simulink library "bh_4bar_SL_LIB"  (R2019a)
settings: Solver=VariableStepAuto  StartTime=0.0  StopTime=10.0  RelTol=1e-3
settings Model: Creator=bhorton  LastModifiedBy=bhorton

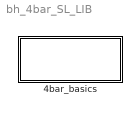
== system bh_4bar_SL_LIB ==
  4bar_basics : Subsystem

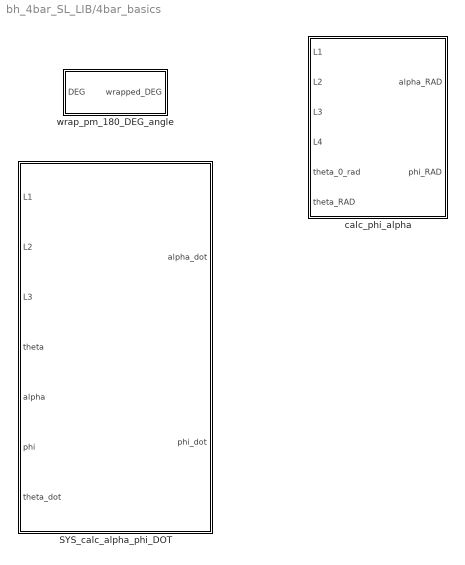
== system bh_4bar_SL_LIB/4bar_basics ==
  SYS_calc_alpha_phi_DOT : Subsystem
  calc_phi_alpha : Subsystem
  wrap_pm_180_DEG_angle : Subsystem

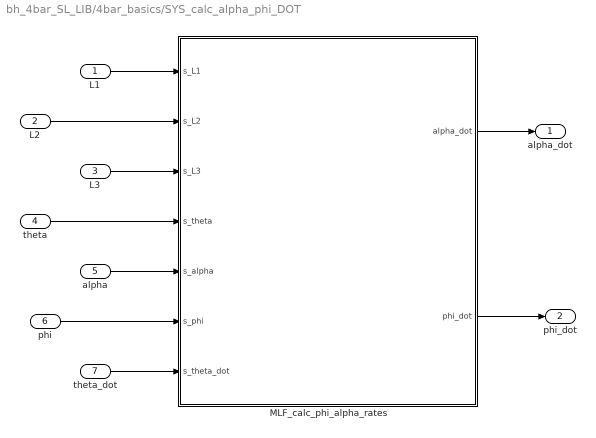
== system bh_4bar_SL_LIB/4bar_basics/SYS_calc_alpha_phi_DOT ==
  L1 : Inport
  L2 : Inport  Port=2
  L3 : Inport  Port=3
  theta : Inport  Port=4
  alpha : Inport  Port=5
  phi : Inport  Port=6
  theta_dot : Inport  Port=7
  MLF_calc_phi_alpha_rates : MATLAB Function  TreatAsAtomicUnit=on
  alpha_dot : Outport
  phi_dot : Outport  Port=2
  wires:
  theta_dot/1 -> MLF_calc_phi_alpha_rates/7(s_theta_dot)
  phi/1 -> MLF_calc_phi_alpha_rates/6(s_phi)
  alpha/1 -> MLF_calc_phi_alpha_rates/5(s_alpha)
  theta/1 -> MLF_calc_phi_alpha_rates/4(s_theta)
  L3/1 -> MLF_calc_phi_alpha_rates/3(s_L3)
  L2/1 -> MLF_calc_phi_alpha_rates/2(s_L2)
  L1/1 -> MLF_calc_phi_alpha_rates/1(s_L1)
  MLF_calc_phi_alpha_rates/2(phi_dot) -> phi_dot/1
  MLF_calc_phi_alpha_rates/1(alpha_dot) -> alpha_dot/1

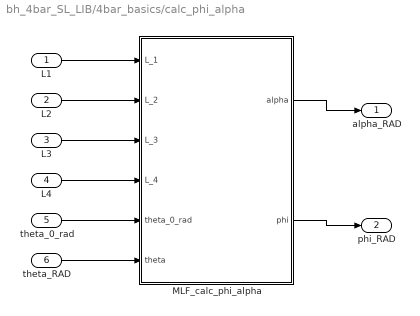
== system bh_4bar_SL_LIB/4bar_basics/calc_phi_alpha ==
  L1 : Inport
  L2 : Inport  Port=2
  L3 : Inport  Port=3
  L4 : Inport  Port=4
  theta_0_rad : Inport  Port=5
  theta_RAD : Inport  Port=6
  MLF_calc_phi_alpha : MATLAB Function  TreatAsAtomicUnit=on
  alpha_RAD : Outport
  phi_RAD : Outport  Port=2
  wires:
  theta_0_rad/1 -> MLF_calc_phi_alpha/5(theta_0_rad)
  MLF_calc_phi_alpha/2(phi) -> phi_RAD/1
  MLF_calc_phi_alpha/1(alpha) -> alpha_RAD/1
  L1/1 -> MLF_calc_phi_alpha/1(L_1)
  L2/1 -> MLF_calc_phi_alpha/2(L_2)
  L3/1 -> MLF_calc_phi_alpha/3(L_3)
  L4/1 -> MLF_calc_phi_alpha/4(L_4)
  theta_RAD/1 -> MLF_calc_phi_alpha/6(theta)

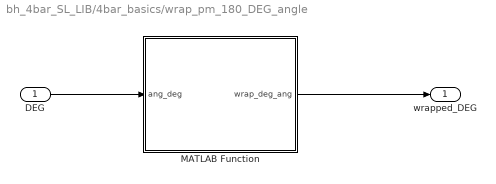
== system bh_4bar_SL_LIB/4bar_basics/wrap_pm_180_DEG_angle ==
  DEG : Inport
  MATLAB Function : MATLAB Function  TreatAsAtomicUnit=on
  wrapped_DEG : Outport
  wires:
  DEG/1 -> MATLAB Function/1(ang_deg)
  MATLAB Function/1(wrap_deg_ang) -> wrapped_DEG/1

== matlab function bh_4bar_SL_LIB/4bar_basics/calc_phi_alpha/MLF_calc_phi_alpha ==
  data: alpha output; L_1 input; phi output; L_2 input; L_3 input; L_4 input; theta_0_rad input; theta input
function [alpha, phi] = calc_phi_alpha(L_1, L_2, L_3, L_4, theta_0_rad, theta)

% Out of the 2 solution scenarios we'll choose the solution that covers the
% situation where phi is POSITIVE when theta==0

[phi_pair_rad, alpha_pair_rad] = bh_angle_calc_util(L_1, L_2, L_3, L_4, theta, "CALC_PHI_AND_ALPHA_VEC");          

[phi_pair_rad_ZERO, alpha_pair_rad_ZERO] = bh_angle_calc_util(L_1, L_2, L_3, L_4, theta_0_rad, "CALC_PHI_AND_ALPHA_VEC");          

if( phi_pair_rad_ZERO(1) >=0 )
  alpha = alpha_pair_rad(1);
  phi   =   phi_pair_rad(1);
else
  alpha = alpha_pair_rad(2);
  phi   =   phi_pair_rad(2);
end
    
% [phi, alpha] = bh_angle_calc_util(L_1, L_2, L_3, L_4, theta, ...
%                 "CALC_PHI_AND_ALPHA_VAL_AND_PHI_IS_POS");
            
end

== matlab function bh_4bar_SL_LIB/4bar_basics/wrap_pm_180_DEG_angle/MATLAB Function ==
  data: ang_deg input; wrap_deg_ang output
function wrap_deg_ang = wrap_to_pm_180(ang_deg)
%#codegen
   wrap_deg_ang = bh_wrap_DEG_angles(ang_deg, "-180_TO_180");
end

== matlab function bh_4bar_SL_LIB/4bar_basics/SYS_calc_alpha_phi_DOT/MLF_calc_phi_alpha_rates ==
  data: alpha_dot output; s_L1 input; phi_dot output; s_L2 input; s_L3 input; s_theta input; s_alpha input; s_phi input; s_theta_dot input
function [alpha_dot, phi_dot ] = ...
       calc_phi_alpha_rates(s_L1, s_L2, s_L3, s_theta, s_alpha, s_phi, s_theta_dot)

   k = 1/( s_L3*s_L2*(sin(s_phi)*cos(s_alpha)   -  cos(s_phi)*sin(s_alpha))  );
       
   tmp_A      =   [-s_L2*cos(s_alpha), -s_L2*sin(s_alpha);
                   -s_L3*cos(s_phi),   -s_L3*sin(s_phi);   ];
               
   tmp_B      =   [ -s_L1*sin(s_theta);
                     s_L1*cos(s_theta); ];
   
   the_jacobs    = k * tmp_A * tmp_B;
   
   dphi_dtheta   =  the_jacobs(1);
   dalpha_dtheta =  the_jacobs(2);   

   phi_dot       = dphi_dtheta   * s_theta_dot;
   alpha_dot     = dalpha_dtheta * s_theta_dot;

end
